simulink model "sync_gazebo"  (R2022a)
settings: Solver=FixedStepAuto  StartTime=0.0  StopTime=10  FixedStep=0.001  RelTol=1e-3
StopFcn:
  | airframe_plot
libraries: robotgazebolib x2, simulink x1, simulink_extras x1
settings Model: Creator=amani  LastModifiedBy=amani

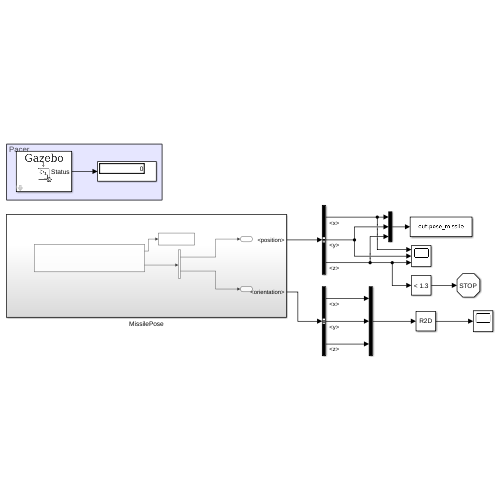
[thumbnail: Simulink's stored preview of the top-level diagram]
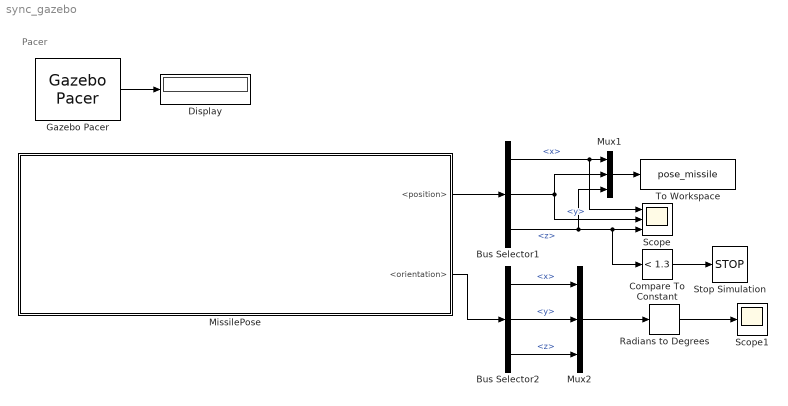
== system sync_gazebo ==
  note: Pacer
  Bus Selector1 : BusSelector  OutputSignals=x,y,z
  Bus Selector2 : BusSelector  OutputSignals=x,y,z
  Compare To Constant : simulink/Logic and Bit Operations/Compare To Constant  relop=<  const=1.3  OutDataTypeStr=boolean
  Display : Display
  Gazebo Pacer : robotgazebolib/Gazebo Pacer  ResetBehavior=Reset Gazebo simulation time and scene  SampleTime=0.001
      settings: SourceProductBaseCode=RO
  MissilePose : Subsystem
  Mux1 : Mux  Inputs=3
  Mux2 : Mux  Inputs=3
  Radians to Degrees : simulink_extras/Transformations/Radians to Degrees
  Scope : Scope  NumInputPorts=3
  Scope1 : Scope
  Stop Simulation : Stop
  To Workspace : ToWorkspace  VariableName=pose_missile  SaveFormat=Structure With Time  SampleTime=-1
  wires:
  Bus Selector1/2 -> Mux1/2, Scope/2  "<y>"
  Bus Selector1/1 -> Scope/1, Mux1/1  "<x>"
  Mux2/1 -> Radians to Degrees/1
  Gazebo Pacer/1 -> Display/1
  Bus Selector2/1 -> Mux2/1  "<x>"
  Bus Selector2/3 -> Mux2/3  "<z>"
  Compare To Constant/1 -> Stop Simulation/1
  Mux1/1 -> To Workspace/1
  Bus Selector2/2 -> Mux2/2  "<y>"
  Bus Selector1/3 -> Compare To Constant/1, Scope/3, Mux1/3  "<z>"
  Radians to Degrees/1 -> Scope1/1
  MissilePose/1(<position>) -> Bus Selector1/1
  MissilePose/2(<orientation>) -> Bus Selector2/1

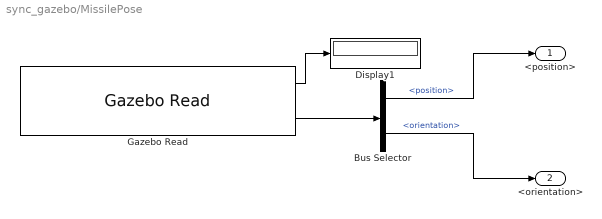
== system sync_gazebo/MissilePose ==
  Bus Selector : BusSelector  OutputSignals=position,orientation
  Display1 : Display
  Gazebo Read : robotgazebolib/Gazebo Read  topicSource=From Gazebo  topic=/gazebo/ground_truth/world_pose/model_missile/base_link  messageType=gazebo_msgs/Pose  sampleTime=0.001
      settings: SourceProductBaseCode=RO
  <position> : Outport
  <orientation> : Outport  Port=2
  wires:
  Gazebo Read/2 -> Bus Selector/1
  Gazebo Read/1 -> Display1/1
  Bus Selector/2 -> <orientation>/1  "<orientation>"
  Bus Selector/1 -> <position>/1  "<position>"
